simulink model "Non_Midline_Y_Connection"  (Simulink 7.5)
settings: Solver=ode15s  StartTime=0.0  StopTime=0.1  RelTol=1e-3
libraries: powerlib x18, powerlib_extras x4
settings Model: Creator=lm  LastModifiedBy=lm

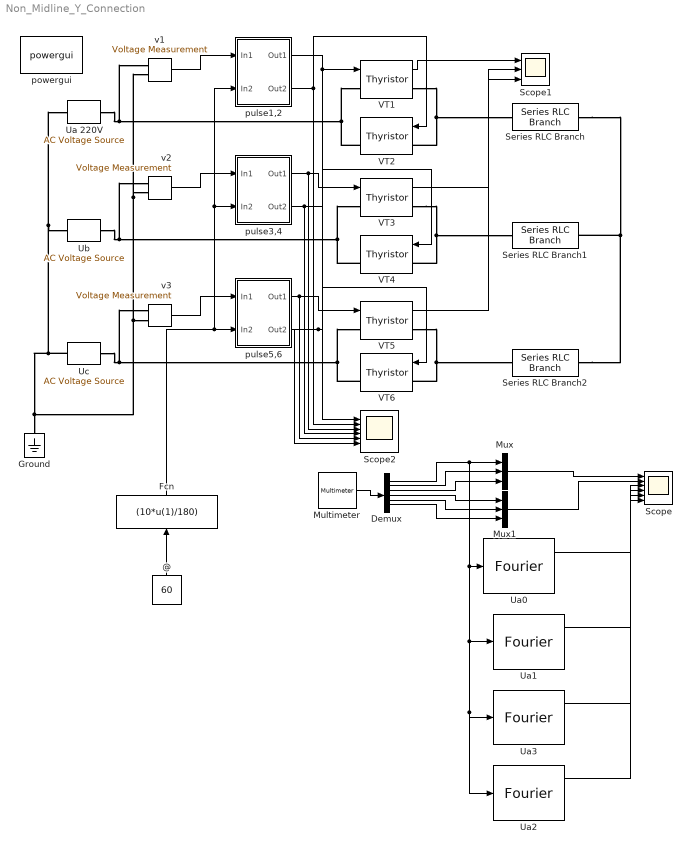
== system Non_Midline_Y_Connection ==
  @ : Constant  Value=60  OutDataType=fixdt(1, 16)  OutScaling=2^0
  Demux : Demux  Outputs=6
  Fcn : Fcn  Expr=(10*u(1)/180)
  Ground : powerlib/Elements/Ground  DialogController=POWERSYS.PowerSysDialog  PhysicalDomain=powersysdomain  SubClassName=unknown  LeftPortType=p1  RightPortType=p1  LConnTagsString=a
  Multimeter : powerlib/Measurements/Multimeter  SystemSampleTime=-1  PhasorSimulation=off  OutputType=Complex  sel=[1 2 3 4 5 6]  L=6  Gain=[1 1 1 1 1 1]  yselected={'Ub: Series RLC Branch','Ub: Series RLC Branch1','Ub: Series RLC Branch2','Ib: Series RLC Branch','Ib: Series RLC Branch1','Ib: Series RLC Branch2'};  PSBOutputType=1  PSBequivalent=0  AxesSetting=[0,0.1,-100,100]  Display=0  SavedBlockNames=-11
  Mux : Mux  Inputs=3
  Mux1 : Mux  Inputs=3
  Scope : Scope  NumInputPorts=6
      settings: YMin=-5~-5~-5~-5~-5~-5  YMax=5~5~5~5~5~5
  Scope1 : Scope  NumInputPorts=3
      settings: YMin=-5~-5~-5  YMax=5~5~5
  Scope2 : Scope  NumInputPorts=6
      settings: TimeRange=0.1  YMin=-0~0~0~0~0~0  YMax=2~2~2~2~2~2  SaveName=ScopeData2
  Series RLC Branch : powerlib/Elements/Series RLC Branch  DialogController=POWERSYS.PowerSysDialog  PhysicalDomain=powersysdomain  SubClassName=unknown  LeftPortType=p1  RightPortType=p1  LConnTagsString=__new0  RConnTagsString=__new0  BranchType=R  Resistance=1  Inductance=1e-3  SetiL0=off  InitialCurrent=0  Capacitance=1e-6  Setx0=off  InitialVoltage=0  Measurements=Branch voltage and current
  Series RLC Branch1 : powerlib/Elements/Series RLC Branch  DialogController=POWERSYS.PowerSysDialog  PhysicalDomain=powersysdomain  SubClassName=unknown  LeftPortType=p1  RightPortType=p1  LConnTagsString=__new0  RConnTagsString=__new0  BranchType=R  Resistance=1  Inductance=1e-3  SetiL0=off  InitialCurrent=0  Capacitance=1e-6  Setx0=off  InitialVoltage=0  Measurements=Branch voltage and current
  Series RLC Branch2 : powerlib/Elements/Series RLC Branch  DialogController=POWERSYS.PowerSysDialog  PhysicalDomain=powersysdomain  SubClassName=unknown  LeftPortType=p1  RightPortType=p1  LConnTagsString=__new0  RConnTagsString=__new0  BranchType=R  Resistance=1  Inductance=1e-3  SetiL0=off  InitialCurrent=0  Capacitance=1e-6  Setx0=off  InitialVoltage=0  Measurements=Branch voltage and current
  Ua 220V : powerlib/Electrical Sources/AC Voltage Source  DialogController=POWERSYS.PowerSysDialog  SystemSampleTime=-1  Amplitude=220  Phase=0  Frequency=50  SampleTime=0  Measurements=None
  Ua0 : powerlib_extras/Measurements/Fourier  DialogController=POWERSYS.PowerSysDialog  SystemSampleTime=-1  f1=50  n=0
  Ua1 : powerlib_extras/Measurements/Fourier  DialogController=POWERSYS.PowerSysDialog  SystemSampleTime=-1  f1=50  n=1
  Ua2 : powerlib_extras/Measurements/Fourier  DialogController=POWERSYS.PowerSysDialog  SystemSampleTime=-1  f1=50  n=2
  Ua3 : powerlib_extras/Measurements/Fourier  DialogController=POWERSYS.PowerSysDialog  SystemSampleTime=-1  f1=50  n=3
  Ub : powerlib/Electrical Sources/AC Voltage Source  DialogController=POWERSYS.PowerSysDialog  SystemSampleTime=-1  Amplitude=220  Phase=-120  Frequency=50  SampleTime=0  Measurements=None
  "Uc " : powerlib/Electrical Sources/AC Voltage Source  DialogController=POWERSYS.PowerSysDialog  SystemSampleTime=-1  Amplitude=220  Phase=-240  Frequency=50  SampleTime=0  Measurements=None
  VT{1..6} (6 alike) : powerlib/Power Electronics/Thyristor  DialogController=POWERSYS.PowerSysDialog  SystemSampleTime=-1  Ron=0.001  Lon=0  Vf=0.8  IC=0  Rs=500  Cs=250e-9  Measurements=on
  powergui : powerlib/powergui  Priority=1  SystemSampleTime=-1  SimulationMode=Discrete  SampleTime=50e-6  frequency=60  SPID=off  DisableSnubberDevices=off  DisableRonSwitches=off  DisableVfSwitches=off  SwTol=0  Interpol=off  frequencyindice=50  echomessages=off  HookPort=off  DisplayEquations=off  FunctionMessages=off  EnableUseOfTLC=off  x0status=blocks  RestoreLinks=warning  ResistiveCurrentMeasurement=off  Ylog=off  Xlog=on  ShowGrid=off  save=off  variable=ZData  ZoomFFT=off  StartTime=0.0  cycles=1  DisplayStyle=1  FreqAxis=off  MaxFrequency=1000  frequencyindicesteady=1  display=off  methode=off
  pulse1,2 : Subsystem
  pulse3,4 : Subsystem
  pulse5,6 : Subsystem
  v1 : powerlib/Measurements/Voltage Measurement  DialogController=POWERSYS.PowerSysDialog  SystemSampleTime=-1  PhasorSimulation=off  OutputType=Complex  PSBequivalent=0
  v2 : powerlib/Measurements/Voltage Measurement  DialogController=POWERSYS.PowerSysDialog  SystemSampleTime=-1  PhasorSimulation=off  OutputType=Complex  PSBequivalent=0
  v3 : powerlib/Measurements/Voltage Measurement  DialogController=POWERSYS.PowerSysDialog  SystemSampleTime=-1  PhasorSimulation=off  OutputType=Complex  PSBequivalent=0
  wires:
  v1/1 -> pulse1,2/1(In1)
  v2/1 -> pulse3,4/1(In1)
  v3/1 -> pulse5,6/1(In1)
  pulse1,2/1(Out1) -> VT1/1, Scope2/1
  pulse1,2/2(Out2) -> VT2/1, Scope2/2
  pulse3,4/1(Out1) -> VT3/1, Scope2/3
  pulse5,6/1(Out1) -> VT5/1, Scope2/5
  pulse3,4/2(Out2) -> VT4/1, Scope2/4
  pulse5,6/2(Out2) -> VT6/1, Scope2/6
  @/1 -> Fcn/1
  Fcn/1 -> pulse5,6/2(In2), pulse3,4/2(In2), pulse1,2/2(In2)
  Multimeter/1 -> Demux/1
  VT1/1 -> Scope1/1
  VT3/1 -> Scope1/2
  VT5/1 -> Scope1/3
  Demux/1 -> Mux/1, Ua0/1, Ua1/1, Ua3/1, Ua2/1
  Demux/2 -> Mux/2
  Demux/3 -> Mux/3
  Demux/4 -> Mux1/1
  Demux/5 -> Mux1/2
  Demux/6 -> Mux1/3
  Mux/1 -> Scope/1
  Mux1/1 -> Scope/2
  Ua0/1 -> Scope/3
  Ua1/1 -> Scope/4
  Ua3/1 -> Scope/5
  Ua2/1 -> Scope/6
  connections:
  "Uc "/LConn1 -- Ub/LConn1 -- Ua 220V/LConn1 -- Ground/LConn1 -- v3/LConn2 -- v1/LConn2 -- v2/LConn2
  Ua 220V/RConn1 -- VT2/RConn1 -- VT1/LConn1 -- v1/LConn1
  VT1/RConn1 -- VT2/LConn1 -- Series RLC Branch/LConn1
  Ub/RConn1 -- VT4/RConn1 -- VT3/LConn1 -- v2/LConn1
  VT3/RConn1 -- VT4/LConn1 -- Series RLC Branch1/LConn1
  VT5/RConn1 -- VT6/LConn1 -- Series RLC Branch2/LConn1
  "Uc "/RConn1 -- VT6/RConn1 -- VT5/LConn1 -- v3/LConn1
  Series RLC Branch/RConn1 -- Series RLC Branch1/RConn1 -- Series RLC Branch2/RConn1

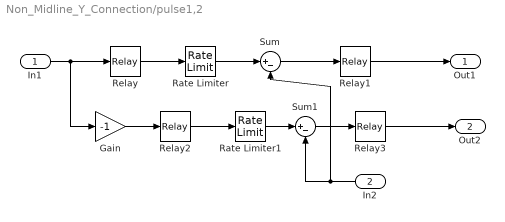
== system Non_Midline_Y_Connection/pulse1,2 ==
  In1 : Inport  OutDataType=fixdt(1, 16)  OutScaling=2^0
  In2 : Inport  Port=2  OutDataType=fixdt(1, 16)  OutScaling=2^0
  Gain : Gain  Gain=-1  ParameterDataType=fixdt(1, 16)  ParameterScaling=2^0  OutDataType=fixdt(1, 16)  OutScaling=2^0
  Rate Limiter : RateLimiter  RisingSlewLimit=1000  FallingSlewLimit=-1e8  SampleTimeMode=inherited
  Rate Limiter1 : RateLimiter  RisingSlewLimit=1000  FallingSlewLimit=-1e9  SampleTimeMode=inherited
  Relay : Relay  OnOutputValue=10  OutDataType=fixdt(1, 16)  OutScaling=2^0
  Relay1 : Relay  OutDataType=fixdt(1, 16)  OutScaling=2^0
  Relay2 : Relay  OnOutputValue=10  OutDataType=fixdt(1, 16)  OutScaling=2^0
  Relay3 : Relay  OutDataType=fixdt(1, 16)  OutScaling=2^0
  Sum : Sum  Inputs=|+-  OutDataType=fixdt(1, 16)  OutScaling=2^0
  Sum1 : Sum  Inputs=|+-  OutDataType=fixdt(1, 16)  OutScaling=2^0
  Out1 : Outport  OutDataType=fixdt(1, 16)  OutScaling=2^0
  Out2 : Outport  Port=2  OutDataType=fixdt(1, 16)  OutScaling=2^0
  wires:
  Rate Limiter/1 -> Sum/1
  Relay/1 -> Rate Limiter/1
  Relay3/1 -> Out2/1
  Sum1/1 -> Relay3/1
  In2/1 -> Sum/2, Sum1/2
  Rate Limiter1/1 -> Sum1/1
  Relay2/1 -> Rate Limiter1/1
  Gain/1 -> Relay2/1
  In1/1 -> Gain/1, Relay/1
  Sum/1 -> Relay1/1
  Relay1/1 -> Out1/1

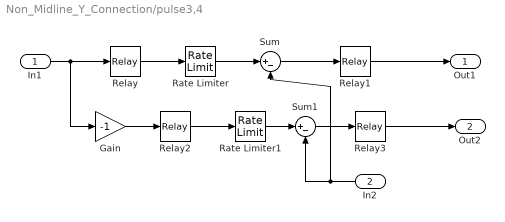
== system Non_Midline_Y_Connection/pulse3,4 ==
  In1 : Inport  OutDataType=fixdt(1, 16)  OutScaling=2^0
  In2 : Inport  Port=2  OutDataType=fixdt(1, 16)  OutScaling=2^0
  Gain : Gain  Gain=-1  ParameterDataType=fixdt(1, 16)  ParameterScaling=2^0  OutDataType=fixdt(1, 16)  OutScaling=2^0
  Rate Limiter : RateLimiter  RisingSlewLimit=1000  FallingSlewLimit=-1e8  SampleTimeMode=inherited
  Rate Limiter1 : RateLimiter  RisingSlewLimit=1000  FallingSlewLimit=-1e9  SampleTimeMode=inherited
  Relay : Relay  OnOutputValue=10  OutDataType=fixdt(1, 16)  OutScaling=2^0
  Relay1 : Relay  OutDataType=fixdt(1, 16)  OutScaling=2^0
  Relay2 : Relay  OnOutputValue=10  OutDataType=fixdt(1, 16)  OutScaling=2^0
  Relay3 : Relay  OutDataType=fixdt(1, 16)  OutScaling=2^0
  Sum : Sum  Inputs=|+-  OutDataType=fixdt(1, 16)  OutScaling=2^0
  Sum1 : Sum  Inputs=|+-  OutDataType=fixdt(1, 16)  OutScaling=2^0
  Out1 : Outport  OutDataType=fixdt(1, 16)  OutScaling=2^0
  Out2 : Outport  Port=2  OutDataType=fixdt(1, 16)  OutScaling=2^0
  wires:
  Relay1/1 -> Out1/1
  Sum/1 -> Relay1/1
  In1/1 -> Relay/1, Gain/1
  Gain/1 -> Relay2/1
  Relay2/1 -> Rate Limiter1/1
  Rate Limiter1/1 -> Sum1/1
  In2/1 -> Sum1/2, Sum/2
  Sum1/1 -> Relay3/1
  Relay3/1 -> Out2/1
  Relay/1 -> Rate Limiter/1
  Rate Limiter/1 -> Sum/1

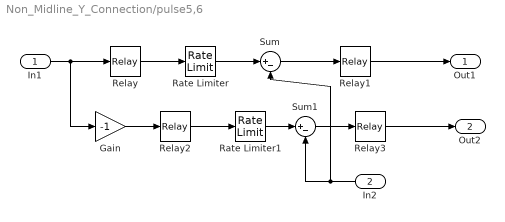
== system Non_Midline_Y_Connection/pulse5,6 ==
  In1 : Inport  OutDataType=fixdt(1, 16)  OutScaling=2^0
  In2 : Inport  Port=2  OutDataType=fixdt(1, 16)  OutScaling=2^0
  Gain : Gain  Gain=-1  ParameterDataType=fixdt(1, 16)  ParameterScaling=2^0  OutDataType=fixdt(1, 16)  OutScaling=2^0
  Rate Limiter : RateLimiter  RisingSlewLimit=1000  FallingSlewLimit=-1e8  SampleTimeMode=inherited
  Rate Limiter1 : RateLimiter  RisingSlewLimit=1000  FallingSlewLimit=-1e9  SampleTimeMode=inherited
  Relay : Relay  OnOutputValue=10  OutDataType=fixdt(1, 16)  OutScaling=2^0
  Relay1 : Relay  OutDataType=fixdt(1, 16)  OutScaling=2^0
  Relay2 : Relay  OnOutputValue=10  OutDataType=fixdt(1, 16)  OutScaling=2^0
  Relay3 : Relay  OutDataType=fixdt(1, 16)  OutScaling=2^0
  Sum : Sum  Inputs=|+-  OutDataType=fixdt(1, 16)  OutScaling=2^0
  Sum1 : Sum  Inputs=|+-  OutDataType=fixdt(1, 16)  OutScaling=2^0
  Out1 : Outport  OutDataType=fixdt(1, 16)  OutScaling=2^0
  Out2 : Outport  Port=2  OutDataType=fixdt(1, 16)  OutScaling=2^0
  wires:
  Rate Limiter/1 -> Sum/1
  Relay/1 -> Rate Limiter/1
  Relay3/1 -> Out2/1
  Sum1/1 -> Relay3/1
  In2/1 -> Sum/2, Sum1/2
  Rate Limiter1/1 -> Sum1/1
  Relay2/1 -> Rate Limiter1/1
  Gain/1 -> Relay2/1
  In1/1 -> Gain/1, Relay/1
  Sum/1 -> Relay1/1
  Relay1/1 -> Out1/1
